simulink model "ik"  (R2017a)
settings: Solver=VariableStepAuto  StartTime=0.0  StopTime=10.0  RelTol=1e-3
settings Model: Creator=Ortix  LastModifiedBy=Ortix

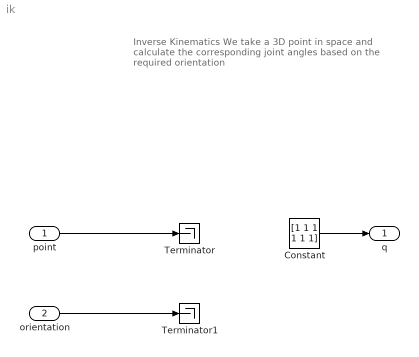
== system ik ==
  note: Inverse Kinematics
      | We take a 3D point in space and calculate the corresponding joint angles based on the required orientation
  point : Inport  PortDimensions=3
  orientation : Inport  Port=2
  Constant : Constant  Value=[1 1 1 1 1 1]
  Terminator : Terminator
  Terminator1 : Terminator
  q : Outport  PortDimensions=6
  wires:
  point/1 -> Terminator/1
  Constant/1 -> q/1
  orientation/1 -> Terminator1/1
